simulink model "Exp_5_single_phase_full_controlled_bridge_rectifer"  (R2021a)
settings: Solver=VariableStepAuto  StartTime=0.0  StopTime=1  RelTol=1e-3
libraries: spsMultimeterLib x4, spsThyristorLib x4, spsACVoltageSourceLib x1, spsCurrentMeasurementLib x1, spsMeanLib x1, spsRMSLib x1, spsSeriesRLCBranchLib x1, spspowerguiLib x1
settings Model: Creator=hp  LastModifiedBy=hp
settings DebuggingCC: UnconnectedInputMsg=none  UnconnectedOutputMsg=none  UnconnectedLineMsg=none

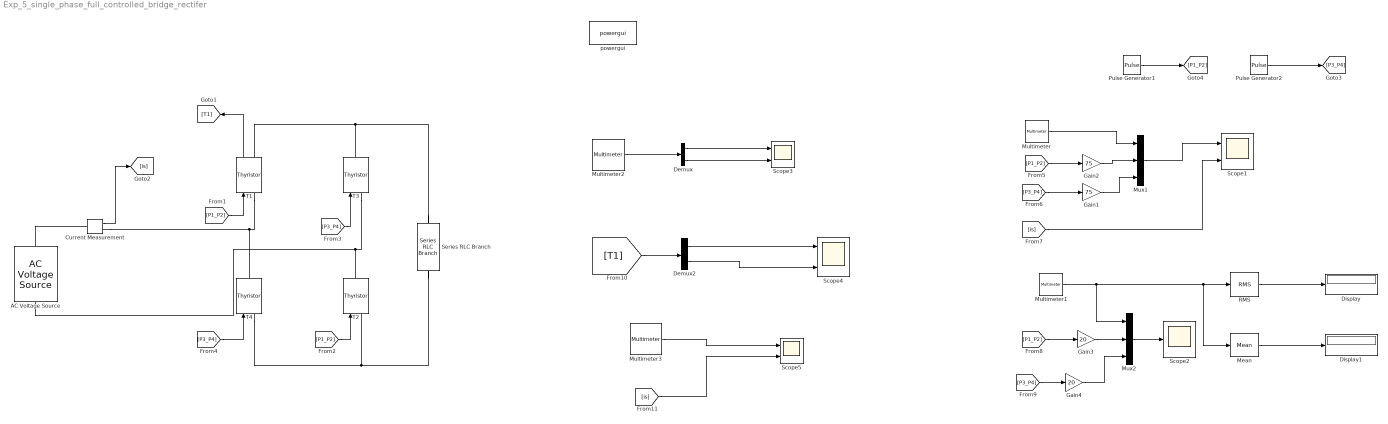
== system Exp_5_single_phase_full_controlled_bridge_rectifer ==
  AC Voltage Source : spsACVoltageSourceLib/AC Voltage Source  Amplitude=100  Phase=0  Frequency=50  SampleTime=0  Measurements=Voltage  BusType=swing  Pref=10e3  Qref=0  Qmin=-inf  Qmax=+inf
  Current Measurement : spsCurrentMeasurementLib/Current Measurement  PhasorSimulation=off  OutputType=Complex  PSBequivalent=0
  Demux : Demux  Outputs=2
  Demux2 : Demux  Outputs=2
  Display : Display
  Display1 : Display
  Gain1 : Gain  Gain=75
  Gain2 : Gain  Gain=75
  Gain3 : Gain  Gain=20
  Gain4 : Gain  Gain=20
  Mean : spsMeanLib/Mean  Freq=50  Vinit=0  Ts=0
  Multimeter : spsMultimeterLib/Multimeter  PhasorSimulation=off  OutputType=Complex  sel=2  L=3  Gain=1  yselected={'Usrc: AC Voltage Source'};  PSBOutputType=1  PSBequivalent=0  AxesSetting=[0,0.1,-100,100]  Display=0  SavedBlockNames=-11
  Multimeter1 : spsMultimeterLib/Multimeter  PhasorSimulation=off  OutputType=Complex  sel=[2 1]  L=3  Gain=[1 1]  yselected={'Usrc: AC Voltage Source','Ub: Series RLC Branch'};  PSBOutputType=1  PSBequivalent=0  AxesSetting=[0,0.1,-100,100]  Display=0  SavedBlockNames=-11
  Multimeter2 : spsMultimeterLib/Multimeter  PhasorSimulation=off  OutputType=Complex  sel=[1 3]  L=3  Gain=[1 1]  yselected={'Ub: Series RLC Branch','Ib: Series RLC Branch'};  PSBOutputType=1  PSBequivalent=0  AxesSetting=[0,0.1,-100,100]  Display=0  SavedBlockNames=-11
  Multimeter3 : spsMultimeterLib/Multimeter  PhasorSimulation=off  OutputType=Complex  sel=2  L=3  Gain=1  yselected={'Usrc: AC Voltage Source'};  PSBOutputType=1  PSBequivalent=0  AxesSetting=[0,0.1,-100,100]  Display=0  SavedBlockNames=-11
  Mux1 : Mux  Inputs=3
  Mux2 : Mux  Inputs=3
  Pulse Generator1 : DiscretePulseGenerator  PulseType=Time based  Period=0.02  PulseWidth=5  PhaseDelay=(0.02/350)*40
  Pulse Generator2 : DiscretePulseGenerator  PulseType=Time based  Period=0.02  PulseWidth=5  PhaseDelay=((0.02/360)*40)+0.01
  RMS : spsRMSLib/RMS  TrueRMS=on  Freq=50  RMSInit=120  Ts=0
  Scope{1,3..5} (4 alike) : Scope  NumInputPorts=2
  Scope2 : Scope
  Series RLC Branch : spsSeriesRLCBranchLib/Series RLC Branch  LConnTagsString=__new0  RConnTagsString=__new0  BranchType=R  Resistance=100  Inductance=80e-3  SetiL0=off  InitialCurrent=0  Capacitance=1e-6  Setx0=off  InitialVoltage=0  Measurements=Branch voltage and current
  T1 : spsThyristorLib/Thyristor  Ron=0.001  Lon=0  Vf=0.8  IC=0  Rs=500  Cs=250e-9  Measurements=on
  T2 : spsThyristorLib/Thyristor  Ron=0.001  Lon=0  Vf=0.8  IC=0  Rs=500  Cs=250e-9  Measurements=off
  T3 : spsThyristorLib/Thyristor  Ron=0.001  Lon=0  Vf=0.8  IC=0  Rs=500  Cs=250e-9  Measurements=off
  T4 : spsThyristorLib/Thyristor  Ron=0.001  Lon=0  Vf=0.8  IC=0  Rs=500  Cs=250e-9  Measurements=off
  powergui : spspowerguiLib/powergui  Priority=1  SimulationMode=Continuous  SampleTime=50e-6  frequency=60  Iterations=50  frequencyindice=50  Pbase=100e6  ErrMax=1e-4  UnitsV=kV  UnitsW=MW  buscounter=0  FunctionMessages=off  echomessages=off  EnableUseOfTLC=off  CurrentSourceSwitches=off  DisableSnubberDevices=off  DisableRonSwitches=off  DisableVfSwitches=off  DisplayEquations=off  AutomaticDiscreteSolvers=off  SolverType=Tustin/Backward Euler (TBE)  Interpol=off  ExternalGateDelay=off  methode=off  Ts=100  x0status=blocks  SPID=on  SwTol=0  HookPort=off  NonlinearTolerance=1e-4  nMaxIteration=100  ContinueOnMaxIteration=off  RestoreLinks=warning  ResistiveCurrentMeasurement=off  Frange=[0:2:500]  Ylog=off  Xlog=on  ShowGrid=off  save=off  variable=ZData  structure=0  ZoomFFT=off  StartTime=0.0  cycles=1  DisplayStyle=1  fundamental=60  FreqAxis=off  MaxFrequency=1000  frequencyindicesteady=1  RmsSteady=1  display=off
  wires:
  [P1_P2] -> T1/1
  [P1_P2] -> T2/1
  [P3_P4] -> T3/1
  [P3_P4] -> T4/1
  T1/1 -> [T1]
  Current Measurement/1 -> [is]
  Pulse Generator1/1 -> [P1_P2]
  Pulse Generator2/1 -> [P3_P4]
  Multimeter/1 -> Mux1/1
  [P1_P2] -> Gain2/1
  Gain2/1 -> Mux1/2
  [P3_P4] -> Gain1/1
  Gain1/1 -> Mux1/3
  Mux1/1 -> Scope1/1
  [is] -> Scope1/2
  [P3_P4] -> Gain4/1
  Gain3/1 -> Mux2/2
  [P1_P2] -> Gain3/1
  Gain4/1 -> Mux2/3
  RMS/1 -> Display/1
  Mean/1 -> Display1/1
  Mux2/1 -> Scope2/1
  Multimeter1/1 -> Mux2/1, Mean/1, RMS/1
  Demux2/1 -> Scope4/1
  Demux2/2 -> Scope4/2
  [T1] -> Demux2/1
  Multimeter2/1 -> Demux/1
  Demux/1 -> Scope3/1
  Demux/2 -> Scope3/2
  Multimeter3/1 -> Scope5/1
  [is] -> Scope5/2
  connections:
  T1/LConn1 -- Current Measurement/RConn1 -- T4/RConn1
  T3/LConn1 -- AC Voltage Source/LConn1 -- T2/RConn1
  T4/LConn1 -- Series RLC Branch/RConn1 -- T2/LConn1
  T3/RConn1 -- Series RLC Branch/LConn1 -- T1/RConn1
  AC Voltage Source/RConn1 -- Current Measurement/LConn1
